simulink model "MotorDCSimulink2"  (R2023a)
settings: Solver=VariableStepAuto  StartTime=0.0  StopTime=10.0  RelTol=1e-3
values from neighbouring files (symbols this model uses):
  beta = 0.0012    [MotorDC.m]
  J = 0.001    [MotorDC.m]
  kt = 0.01    [MotorDC.m]
  kv = 0.01    [MotorDC.m]
  L = 0.023    [MotorDC.m]
  R = 2    [MotorDC.m]
settings Model: Creator=mluser  LastModifiedBy=mluser
settings OptimizationCC: ReuseModelBlockBuffer=off

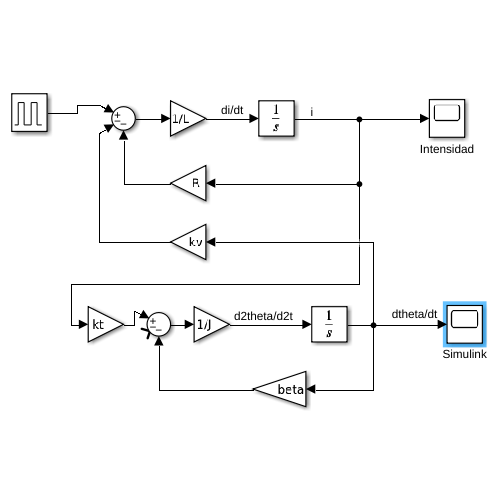
[thumbnail: Simulink's stored preview of the top-level diagram]
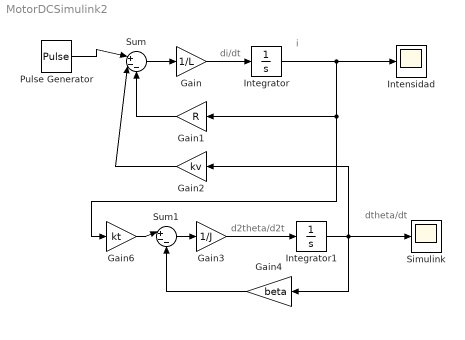
== system MotorDCSimulink2 ==
  note: i
  note: di/dt
  note: d2theta/d2t
  note: dtheta/dt
  Gain : Gain  Gain=1/L
  Gain1 : Gain  Gain=R
  Gain2 : Gain  Gain=kv
  Gain3 : Gain  Gain=1/J
  Gain4 : Gain  Gain=beta
  Gain6 : Gain  Gain=kt
  Integrator : Integrator
  Integrator1 : Integrator
  Intensidad : Scope
  Pulse Generator : DiscretePulseGenerator  PulseType=Time based  Amplitude=24  Period=1/20000  PulseWidth=25
  Simulink : Scope
  Sum : Sum  Inputs=|+--
  Sum1 : Sum  Inputs=|+--
  wires:
  Integrator/1 -> Gain6/1, Gain1/1, Intensidad/1
  Sum/1 -> Gain/1
  Gain/1 -> Integrator/1
  Gain1/1 -> Sum/3
  Gain2/1 -> Sum/2
  Gain3/1 -> Integrator1/1
  Gain6/1 -> Sum1/1
  Sum1/1 -> Gain3/1
  Integrator1/1 -> Gain2/1, Gain4/1, Simulink/1
  Gain4/1 -> Sum1/3
  Pulse Generator/1 -> Sum/1
